simulink model "control_sys"  (R2025b)
settings: Solver=VariableStepAuto  StartTime=0.0  StopTime=10.0  RelTol=1e-3
settings Model: Creator=nolan  LastModifiedBy=nolan

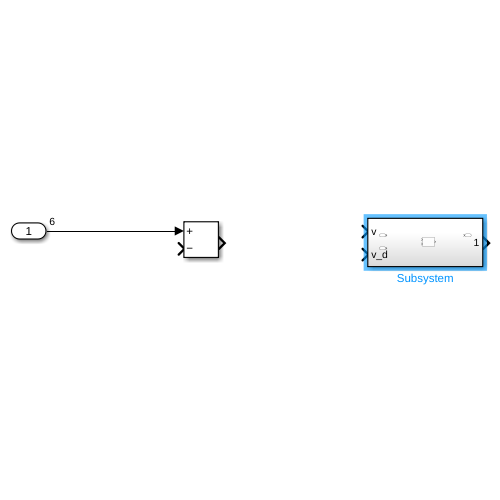
[thumbnail: Simulink's stored preview of the top-level diagram]
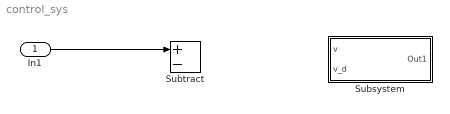
== system control_sys ==
  In1 : Inport  PortDimensions=6
  Subsystem : Subsystem
  Subtract : Sum  Inputs=+-
  wires:
  In1/1 -> Subtract/1

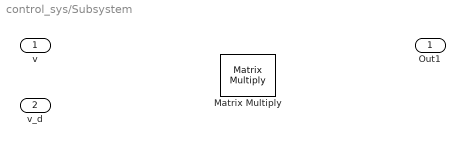
== system control_sys/Subsystem ==
  v : Inport  PortDimensions=6
  v_d : Inport  Port=2
  Matrix Multiply : Product  Multiplication=Matrix(*)
  Out1 : Outport
